simulink model "inductionmotor"  (R2021a)
settings: Solver=VariableStepAuto  StartTime=0.0  StopTime=10.0  RelTol=1e-3
undefined symbols (not defined in the file): Ion, Lithium
libraries: spsIGBTDiodeLib x6, spsSeriesRLCBranchLib x5, simulink x4, spsVoltageMeasurementLib x2, pid_lib x1, spsAsynchronousMachineSIUnitsLib x1, spsPWMGeneratorDCDCLib x1, spsPVArrayLib x1, spsBatteryLib x1, spsCurrentMeasurementLib x1, spsDiodeLib x1, spsMosfetLib x1
settings Model: Creator=Gue$t  LastModifiedBy=Gue$t

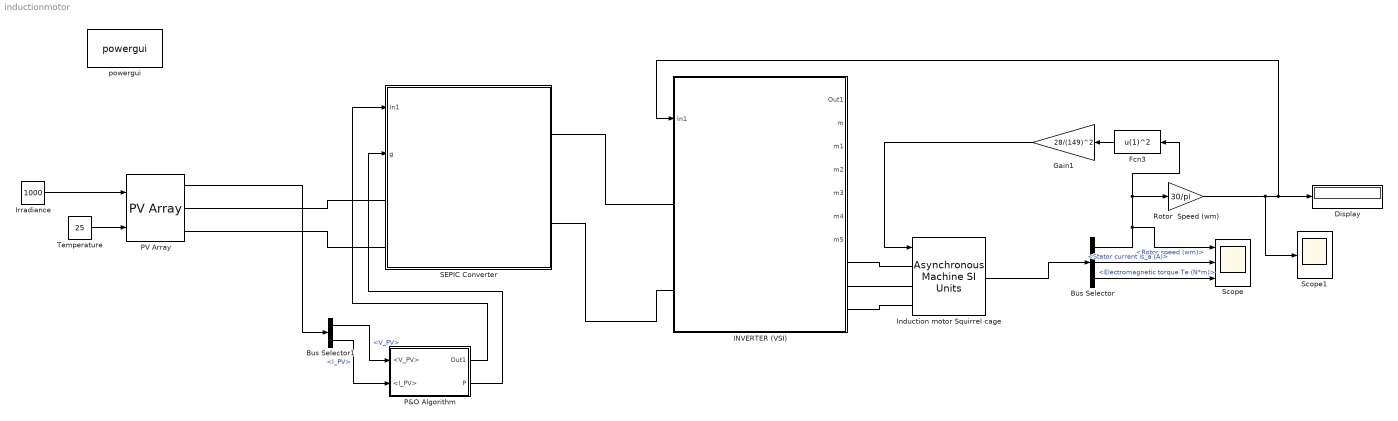
== system inductionmotor ==
  Bus Selector : BusSelector  OutputSignals=Mechanical.Rotor speed (wm),Stator measurements.Stator current is_a (A),Mechanical.Electromagnetic torque Te (N*m)
  Bus Selector1 : BusSelector  OutputSignals=V_PV,I_PV
  Display : Display
  Fcn3 : Fcn  Expr=u(1)^2
  Gain1 : Gain  Gain=28/(149)^2
  INVERTER (VSI) : Subsystem
  Induction motor Squirrel cage : spsAsynchronousMachineSIUnitsLib/Asynchronous Machine SI Units  RotorType=Squirrel-cage  PresetModel="01:  5 HP   460 V 60Hz 1750 RPM"  MechanicalLoad=Torque Tm  ShowDetailedParameters=on  ReferenceFrame=Rotor  Units=SI  MeasurementBus=off  NominalParameters=[3730 460 60]  VoltageRatio=1  Stator=[1.115 0.005974]  Rotor=[1.083 0.005974]  Cage1=[0.4155 0.002066]  Cage2=[0.4168 0.0003495]  Lm=0.2037  Mechanical=[0.02 0.005752 2]  PolePairs=2  InitialConditions=[1 0 0 0 0 0 0 0]  SimulateSaturation=off  Saturation=[14.03593122, 27.81365428, 53.79336849, 72.68890987, 97.98006896, 148.6815601, 215.7428561, 302.9841135, 428.7778367 ; 230, 322, 414, 460, 506, 552, 598, 644, 690]  LoadFlowParameters=1492000  TsPowergui=0  TsBlock=-1  IterativeModel=Trapezoidal non iterative  IterativeDiscreteModel=Trapezoidal non iterative  Pmec=1.492e+006
  Irradiance : Constant  Value=1000
  P&O Algorithm : Subsystem
  PV Array : spsPVArrayLib/PV Array  Npar=2  Nser=3  PlotType=array @ 1000 W/m2 & specified temperatures  S_vec="[ 1000  500  100 ]"  Temp_C_vec="[ 45 25  ]"  ModuleName=User-defined  PlotWhenSelected=off  Pm=224.757  Ncell=60  Voc=41.79  Isc=7.13  Vm=33.9  Im=6.63  beta_Voc_pc=-0.36099  alpha_Isc_pc=0.102  beta_Voc=-0.15086  alpha_Isc=0.0072726  IL=7.142  I0=2.6501e-10  nI=1.1299  Rsh=247.0314  Rs=0.41409  RobustModel=off  RobustCellTemperature=313.3991  BAL=on  Tc=1e-6  Tfilter=5e-5
  Rotor  Speed (wm) : Gain  Gain=30/pi
  SEPIC Converter : Subsystem
  Scope : Scope  NumInputPorts=3
  Scope1 : Scope
  Temperature : Constant  Value=25
  powergui : spspowerguiLib/powergui  Priority=1  SimulationMode=Discrete  SampleTime=1e-6  frequency=60  Iterations=50  frequencyindice=60  Pbase=100e6  ErrMax=1e-4  UnitsV=kV  UnitsW=MW  buscounter=0  FunctionMessages=off  echomessages=off  EnableUseOfTLC=off  CurrentSourceSwitches=off  DisableSnubberDevices=off  DisableRonSwitches=off  DisableVfSwitches=off  DisplayEquations=off  AutomaticDiscreteSolvers=off  SolverType=Tustin/Backward Euler (TBE)  Interpol=off  ExternalGateDelay=off  methode=off  Ts=100  x0status=blocks  SPID=on  SwTol=0  HookPort=off  NonlinearTolerance=0  nMaxIteration=15  ContinueOnMaxIteration=off  RestoreLinks=warning  ResistiveCurrentMeasurement=off  Frange=[0:2:500]  Ylog=off  Xlog=on  ShowGrid=off  save=off  variable=ZData  structure=0  ZoomFFT=off  StartTime=0.0  cycles=1  DisplayStyle=1  fundamental=60  FreqAxis=off  MaxFrequency=1000  frequencyindicesteady=1  RmsSteady=1  display=off
  wires:
  Bus Selector1/2 -> P&O Algorithm/2(<I_PV>)  "<I_PV>"
  PV Array/1 -> Bus Selector1/1
  Irradiance/1 -> PV Array/1
  Bus Selector1/1 -> P&O Algorithm/1(<V_PV>)  "<V_PV>"
  P&O Algorithm/2(P) -> SEPIC Converter/2(g)
  P&O Algorithm/1(Out1) -> SEPIC Converter/1(In1)
  Temperature/1 -> PV Array/2
  Bus Selector/3 -> Scope/3  "<Electromagnetic torque Te (N*m)>"
  Fcn3/1 -> Gain1/1
  Gain1/1 -> Induction motor Squirrel cage/1
  Induction motor Squirrel cage/1 -> Bus Selector/1
  Bus Selector/1 -> Fcn3/1, Rotor  Speed (wm)/1, Scope/1  "<Rotor speed (wm)>"
  Rotor  Speed (wm)/1 -> INVERTER (VSI)/1(In1), Display/1, Scope1/1
  Bus Selector/2 -> Scope/2  "<Stator current is_a (A)>"
  connections:
  PV Array/RConn1 -- SEPIC Converter/LConn1
  PV Array/RConn2 -- SEPIC Converter/LConn2
  SEPIC Converter/RConn2 -- INVERTER (VSI)/LConn2
  SEPIC Converter/RConn1 -- INVERTER (VSI)/LConn1
  Induction motor Squirrel cage/LConn1 -- INVERTER (VSI)/RConn1
  Induction motor Squirrel cage/LConn2 -- INVERTER (VSI)/RConn2
  Induction motor Squirrel cage/LConn3 -- INVERTER (VSI)/RConn3

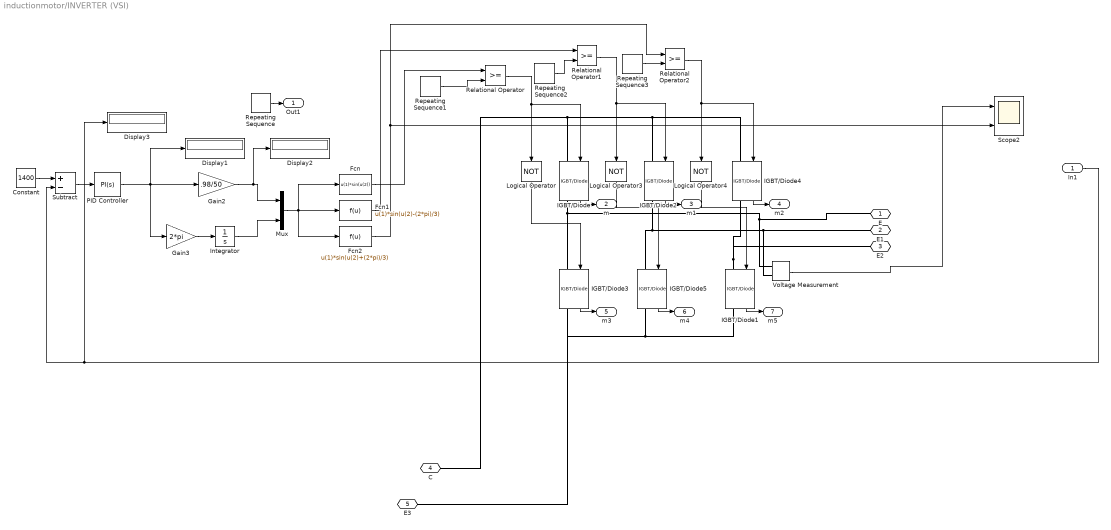
== system inductionmotor/INVERTER (VSI) ==
  In1 : Inport
  Constant : Constant  Value=1400
  Display1 : Display
  Display2 : Display
  Display3 : Display
  Fcn : Fcn  Expr=u(1)*sin(u(2))
  Fcn1 : Fcn  Expr=u(1)*sin(u(2)-(2*pi)/3)
  Fcn2 : Fcn  Expr=u(1)*sin(u(2)+(2*pi)/3)
  Gain2 : Gain  Gain=.98/50
  Gain3 : Gain  Gain=2*pi
  IGBT/Diode{,1..5} (6 alike) : spsIGBTDiodeLib/IGBT//Diode  Ron=1e-3  Rs=1e5  Cs=inf  Measurements=on
  Integrator : Integrator
  Logical Operator : Logic  Operator=NOT  AllPortsSameDT=off  OutDataTypeStr=boolean
  Logical Operator3 : Logic  Operator=NOT  AllPortsSameDT=off  OutDataTypeStr=boolean
  Logical Operator4 : Logic  Operator=NOT  AllPortsSameDT=off  OutDataTypeStr=boolean
  Mux : Mux  Inputs=2
  PID Controller : pid_lib/PID Controller  Controller=PI  Form=Parallel  TimeDomain=Continuous-time  UseExternalTs=off  SampleTime=-1  IntegratorMethod=Forward Euler  FilterMethod=Forward Euler  ControllerParametersSource=internal  P=.0001  I=.1  D=0  UseFilter=on  N=100  TunerSelectOption=Transfer Function Based (PID Tuner App)  InitialConditionSource=internal  InitialConditionForIntegrator=0  InitialConditionForFilter=0  DifferentiatorICPrevScaledInput=0  ExternalReset=none  TrackingMode=off  Kt=1  LimitOutput=on  SatLimitsSource=internal  UpperSaturationLimit=50  LowerSaturationLimit=-50  LinearizeAsGain=on  AntiWindupMode=clamping  Kb=1  POutMin=[]  POutMax=[]  IOutMin=[]  IOutMax=[]  DOutMin=[]  DOutMax=[]  NOutMin=[]  NOutMax=[]  SumOutMin=[]  SumOutMax=[]  SaturationOutMin=[]  SaturationOutMax=[]  PParamMin=[]  PParamMax=[]  IParamMin=[]  IParamMax=[]  DParamMin=[]  DParamMax=[]  NParamMin=[]  NParamMax=[]  KbParamMin=[]  KbParamMax=[]  KtParamMin=[]  KtParamMax=[]  KbOutMin=[]  KbOutMax=[]  KtOutMin=[]  KtOutMax=[]  IntegratorOutMin=[]  IntegratorOutMax=[]  FilterOutMin=[]  FilterOutMax=[]  SumI1OutMin=[]  SumI1OutMax=[]  SumI2OutMin=[]  SumI2OutMax=[]  SumI3OutMin=[]  SumI3OutMax=[]  SumI4OutMin=[]  SumI4OutMax=[]  SumDOutMin=[]  SumDOutMax=[]  DifferentiatorOutMin=[]  DifferentiatorOutMax=[]  FilterDiffOutCoefMin=[]  FilterDiffOutCoefMax=[]  ReciprocalOutMin=[]  ReciprocalOutMax=[]  SumDenOutMin=[]  SumDenOutMax=[]  SumNumOutMin=[]  SumNumOutMax=[]  DivideOutMin=[]  DivideOutMax=[]  UdiffTsProdOutMin=[]  UdiffTsProdOutMax=[]  NTsProdOutMin=[]  NTsProdOutMax=[]  UintegralTsProdOutMin=[]  UintegralTsProdOutMax=[]  UngainTsProdOutMin=[]  UngainTsProdOutMax=[]  IntegratorContinuousStateAttributes=''  IntegratorStateMustResolveToSignalObject=off  IntegratorRTWStateStorageClass=Auto  FilterContinuousStateAttributes=''  FilterStateMustResolveToSignalObject=off  FilterRTWStateStorageClass=Auto  ParallelPVariant=InternalParameters  IdealPVariant=Disabled  IVariant=InternalParameters  DVariant=Disabled  IntegratorVariant=Continuous  SatVariant=Enabled  AWVariant=ContClampingParallel  PCopyVariant=Disabled  TRVariant=Disabled  FdbkBlocksVariant=Forward  IdealPFdbkVariant=Disabled  SatFdbkVariant=Disabled  DerivativeFilterVariant=Disabled  NVariant=Disabled  NCopyVariant=Disabled_SignalSpec  FilterICVariant=Disabled  IntegratorICVariant=InternalICs  ExternalResetVariant=Disabled  TRSumVariant=Passthrough  SumFdbkVariant=Disabled  SumVariant=Sum_PI  TsampFilterVariant=InternalTs  TsampNgainVariant=Passthrough  TsampIntegralVariant=Passthrough  ExternalSaturationOutDataTypeStr=Inherit: Same as second input
  Relational Operator : RelationalOperator  OutDataTypeStr=boolean  RndMeth=Simplest
  Relational Operator1 : RelationalOperator  OutDataTypeStr=boolean  RndMeth=Simplest
  Relational Operator2 : RelationalOperator  OutDataTypeStr=boolean  RndMeth=Simplest
  Repeating Sequence : simulink/Sources/Repeating Sequence  rep_seq_t=[0 .1 10]  rep_seq_y=[0 50 50]
  Repeating Sequence1 : simulink/Sources/Repeating Sequence  rep_seq_t=[0 (1/5000)/4 (1/5000)/2 (3/5000)/4 1/5000]  rep_seq_y=[0 1 0 -1 0]
  Repeating Sequence2 : simulink/Sources/Repeating Sequence  rep_seq_t=[0 (1/5000)/4 (1/5000)/2 (3/5000)/4 1/5000]  rep_seq_y=[0 1 0 -1 0]
  Repeating Sequence3 : simulink/Sources/Repeating Sequence  rep_seq_t=[0 (1/5000)/4 (1/5000)/2 (3/5000)/4 1/5000]  rep_seq_y=[0 1 0 -1 0]
  Scope2 : Scope  NumInputPorts=2
  Subtract : Sum  Inputs=+-
  Voltage Measurement : spsVoltageMeasurementLib/Voltage Measurement  PhasorSimulation=off  OutputType=Complex  PSBequivalent=0
  E : PMIOPort  Side=Right
  E1 : PMIOPort  Port=2  Side=Right
  E2 : PMIOPort  Port=3  Side=Right
  C : PMIOPort  Port=4  Side=Left
  E3 : PMIOPort  Port=5  Side=Left
  Out1 : Outport
  m : Outport  Port=2
  m1 : Outport  Port=3
  m2 : Outport  Port=4
  m3 : Outport  Port=5
  m4 : Outport  Port=6
  m5 : Outport  Port=7
  wires:
  Repeating Sequence/1 -> Out1/1
  Logical Operator/1 -> IGBT/Diode3/1
  Repeating Sequence1/1 -> Relational Operator/2
  Repeating Sequence3/1 -> Relational Operator2/2
  Integrator/1 -> Mux/2
  Repeating Sequence2/1 -> Relational Operator1/2
  Fcn/1 -> Relational Operator/1
  Relational Operator1/1 -> IGBT/Diode2/1, Logical Operator3/1
  Relational Operator2/1 -> IGBT/Diode4/1, Logical Operator4/1
  In1/1 -> Subtract/2, Display3/1
  Logical Operator4/1 -> IGBT/Diode1/1
  Fcn2/1 -> Relational Operator2/1, Scope2/2
  IGBT/Diode3/1 -> m3/1
  Logical Operator3/1 -> IGBT/Diode5/1
  Gain2/1 -> Display2/1, Mux/1
  Mux/1 -> Fcn2/1, Fcn/1, Fcn1/1
  Fcn1/1 -> Relational Operator1/1
  Voltage Measurement/1 -> Scope2/1
  Relational Operator/1 -> IGBT/Diode/1, Logical Operator/1
  Gain3/1 -> Integrator/1
  Subtract/1 -> PID Controller/1
  PID Controller/1 -> Display1/1, Gain3/1, Gain2/1
  Constant/1 -> Subtract/1
  IGBT/Diode4/1 -> m2/1
  IGBT/Diode1/1 -> m5/1
  IGBT/Diode/1 -> m/1
  IGBT/Diode2/1 -> m1/1
  IGBT/Diode5/1 -> m4/1
  connections:
  IGBT/Diode1/RConn1 -- E3/RConn1 -- IGBT/Diode3/RConn1 -- IGBT/Diode5/RConn1
  IGBT/Diode/LConn1 -- C/RConn1 -- IGBT/Diode4/LConn1 -- IGBT/Diode2/LConn1
  IGBT/Diode1/LConn1 -- E2/RConn1 -- IGBT/Diode4/RConn1
  Voltage Measurement/LConn1 -- IGBT/Diode/RConn1 -- IGBT/Diode3/LConn1 -- E/RConn1
  Voltage Measurement/LConn2 -- E1/RConn1 -- IGBT/Diode2/RConn1 -- IGBT/Diode5/LConn1

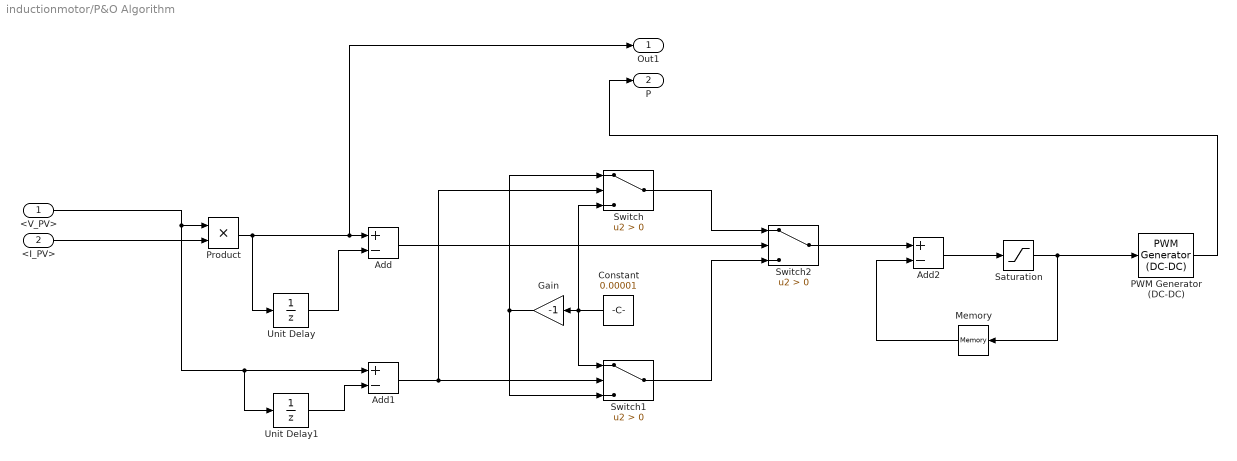
== system inductionmotor/P&O Algorithm ==
  <V_PV> : Inport
  <I_PV> : Inport  Port=2
  Add : Sum  Inputs=+-
  Add1 : Sum  Inputs=+-
  Add2 : Sum  Inputs=+-
  Constant : Constant  Value=0.00001
  Gain : Gain  Gain=-1
  Memory : Memory
  PWM Generator (DC-DC) : spsPWMGeneratorDCDCLib/PWM Generator (DC-DC)  Fsw=50  Ts=0
      link override Sawtooth Generator/Model/Hit  Crossing: HitCrossingOffset=0.001
  Product : Product
  Saturation : Saturate
  Switch : Switch  Criteria=u2 > Threshold
  Switch1 : Switch  Criteria=u2 > Threshold
  Switch2 : Switch  Criteria=u2 > Threshold
  Unit Delay : UnitDelay  SampleTime=-1  HasFrameUpgradeWarning=on
  Unit Delay1 : UnitDelay  SampleTime=-1  HasFrameUpgradeWarning=on
  Out1 : Outport
  P : Outport  Port=2
  wires:
  Add1/1 -> Switch/2, Switch1/2
  Constant/1 -> Switch1/1, Switch/3, Gain/1
  Product/1 -> Out1/1, Add/1, Unit Delay/1
  Gain/1 -> Switch1/3, Switch/1
  Switch/1 -> Switch2/1
  PWM Generator (DC-DC)/1 -> P/1
  Switch2/1 -> Add2/1
  Add/1 -> Switch2/2
  Switch1/1 -> Switch2/3
  Saturation/1 -> Memory/1, PWM Generator (DC-DC)/1
  <V_PV>/1 -> Add1/1, Unit Delay1/1, Product/1
  Unit Delay1/1 -> Add1/2
  Add2/1 -> Saturation/1
  Unit Delay/1 -> Add/2
  Memory/1 -> Add2/2
  <I_PV>/1 -> Product/2

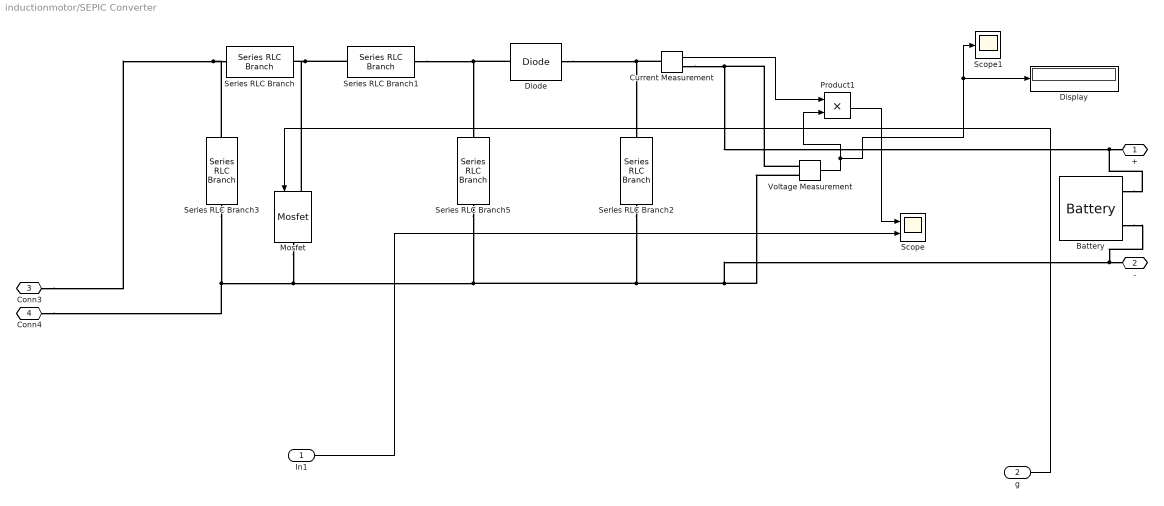
== system inductionmotor/SEPIC Converter ==
  In1 : Inport
  g : Inport  Port=2
  Battery : spsBatteryLib/Battery  BatType=Lithium-Ion  ShowTempParam=off  ThermalPreset=no  ShowAgeParam=off  NomV=350  NomQ=5.4  SOC=100  Batt_Tr=30  PresetModel=on  MaxQ=5.4  MinV=262.5  FullV=407.3955  Dis_rate=2.3478  R=0.64815  Normal_OP=4.8835  expZone="[378.135     0.2653043]"  current=[6.5 13 32.5]  Units=Time  Tci=20  NomT=20  T2=-30  MaxQ2=4.8  FullV2=7.1  Normal_OP2=5.655  expZone2="[6.58           1]"  Rca=0.6  ti=2000  Dp=0  Neq0=0  Tsim=1e6  Ta1=25  Qeol=5.4*0.9  Reol=0.013333*1.2  Char_age=[2.3478, 3]  Dis_age=[2.3478, 10]  N1=1500  N2=10500  N3=1000  N4=1400  Ta2=45  N5=950
  Current Measurement : spsCurrentMeasurementLib/Current Measurement  PhasorSimulation=off  OutputType=Complex  PSBequivalent=0
  Diode : spsDiodeLib/Diode  Ron=0.001  Lon=0  Vf=0.8  IC=0  UseSnubber=0  Rs=500  Cs=250e-9  Measurements=off
  Display : Display
  Mosfet : spsMosfetLib/Mosfet  Ron=0.1  Lon=0  Rd=0.01  Vfd=0  IC=0  Rs=1e5  Cs=inf  Measurements=off
  Product1 : Product
  Scope : Scope  NumInputPorts=2
  Scope1 : Scope
  Series RLC Branch : spsSeriesRLCBranchLib/Series RLC Branch  LConnTagsString=__new0  RConnTagsString=__new0  BranchType=L  Resistance=1  Inductance=2.12e-3  SetiL0=off  InitialCurrent=0  Capacitance=1e-6  Setx0=off  InitialVoltage=0  Measurements=None
  Series RLC Branch1 : spsSeriesRLCBranchLib/Series RLC Branch  LConnTagsString=__new0  RConnTagsString=__new0  BranchType=C  Resistance=1  Inductance=1e-3  SetiL0=off  InitialCurrent=0  Capacitance=1100e-6  Setx0=off  InitialVoltage=0  Measurements=None
  Series RLC Branch2 : spsSeriesRLCBranchLib/Series RLC Branch  LConnTagsString=__new0  RConnTagsString=__new0  BranchType=C  Resistance=1  Inductance=1e-3  SetiL0=off  InitialCurrent=0  Capacitance=1100e-6  Setx0=off  InitialVoltage=0  Measurements=None
  Series RLC Branch3 : spsSeriesRLCBranchLib/Series RLC Branch  LConnTagsString=__new0  RConnTagsString=__new0  BranchType=C  Resistance=1  Inductance=1e-3  SetiL0=off  InitialCurrent=0  Capacitance=1100e-6  Setx0=off  InitialVoltage=0  Measurements=None
  Series RLC Branch5 : spsSeriesRLCBranchLib/Series RLC Branch  LConnTagsString=__new0  RConnTagsString=__new0  BranchType=L  Resistance=1  Inductance=2.12e-3  SetiL0=off  InitialCurrent=0  Capacitance=1e-6  Setx0=off  InitialVoltage=0  Measurements=None
  Voltage Measurement : spsVoltageMeasurementLib/Voltage Measurement  PhasorSimulation=off  OutputType=Complex  PSBequivalent=0
  + : PMIOPort  Side=Right
  - : PMIOPort  Port=2  Side=Right
  Conn3 : PMIOPort  Port=3  Side=Left
  Conn4 : PMIOPort  Port=4  Side=Left
  wires:
  Voltage Measurement/1 -> Product1/2, Scope1/1, Display/1
  Product1/1 -> Scope/1
  g/1 -> Mosfet/1
  Current Measurement/1 -> Product1/1
  In1/1 -> Scope/2
  connections:
  Series RLC Branch1/LConn1 -- Mosfet/LConn1 -- Series RLC Branch/RConn1
  Current Measurement/LConn1 -- Diode/RConn1 -- Series RLC Branch2/LConn1
  Series RLC Branch3/LConn1 -- Series RLC Branch/LConn1 -- Conn3/RConn1
  Series RLC Branch1/RConn1 -- Diode/LConn1 -- Series RLC Branch5/LConn1
  Current Measurement/RConn1 -- Voltage Measurement/LConn1 -- Battery/LConn1 -- +/RConn1
  Mosfet/RConn1 -- Series RLC Branch5/RConn1 -- Voltage Measurement/LConn2 -- Battery/LConn2 -- -/RConn1 -- Series RLC Branch2/RConn1 -- Series RLC Branch3/RConn1 -- Conn4/RConn1
